simulink model "PI_controller_differentKP_KI"  (R2023b)
settings: Solver=VariableStepAuto  StartTime=0.0  StopTime=10.0  RelTol=1e-3
settings Model: Creator=ascom  LastModifiedBy=ascom

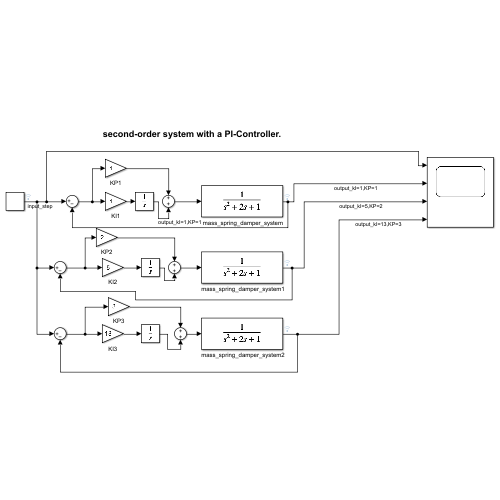
[thumbnail: Simulink's stored preview of the top-level diagram]
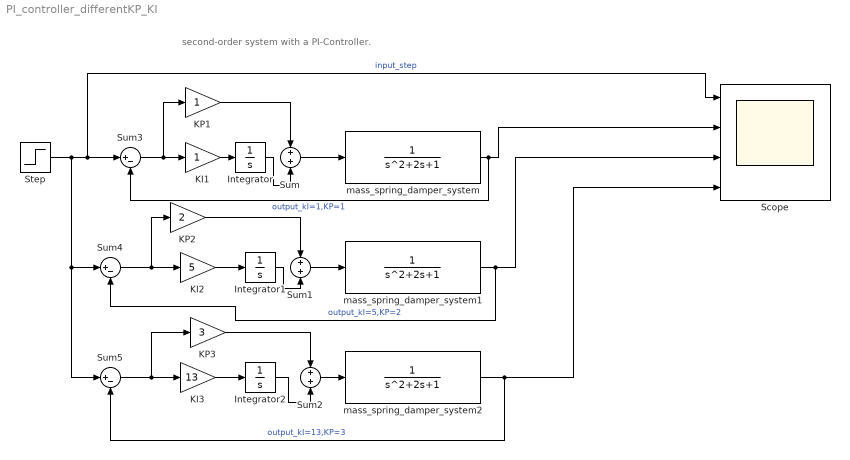
== system PI_controller_differentKP_KI ==
  note: second-order system with a PI-Controller.
  " mass_spring_damper_system" : TransferFcn
  " mass_spring_damper_system1" : TransferFcn
  " mass_spring_damper_system2" : TransferFcn
  Integrator : Integrator
  Integrator1 : Integrator
  Integrator2 : Integrator
  KI1 : Gain
  KI2 : Gain  Gain=5
  KI3 : Gain  Gain=13
  KP1 : Gain
  KP2 : Gain  Gain=2
  KP3 : Gain  Gain=3
  Scope : Scope  NumInputPorts=4
  Step : Step  SampleTime=0
  Sum : Sum
  Sum1 : Sum
  Sum2 : Sum
  Sum3 : Sum  Inputs=|+-
  Sum4 : Sum  Inputs=|+-
  Sum5 : Sum  Inputs=|+-
  wires:
  KI3/1 -> Integrator2/1
  " mass_spring_damper_system2"/1 -> Scope/4, Sum5/2  "output_kI=13,KP=3"
  " mass_spring_damper_system1"/1 -> Sum4/2, Scope/3  "output_kI=5,KP=2"
  KI1/1 -> Integrator/1
  KI2/1 -> Integrator1/1
  KP1/1 -> Sum/1
  Sum/1 -> " mass_spring_damper_system"/1
  Integrator/1 -> Sum/2
  Sum1/1 -> " mass_spring_damper_system1"/1
  KP2/1 -> Sum1/1
  Integrator1/1 -> Sum1/2
  Sum2/1 -> " mass_spring_damper_system2"/1
  KP3/1 -> Sum2/1
  Integrator2/1 -> Sum2/2
  " mass_spring_damper_system"/1 -> Scope/2, Sum3/2  "output_kI=1,KP=1"
  Sum5/1 -> KP3/1, KI3/1
  Sum4/1 -> KP2/1, KI2/1
  Sum3/1 -> KP1/1, KI1/1
  Step/1 -> Sum5/1, Sum4/1, Scope/1, Sum3/1  "input_step"
